simulink model "hopperDesign"  (R2023b)
settings: Solver=VariableStepAuto  StartTime=0.0  StopTime=10.0  RelTol=1e-3
settings Model: Creator=adrnf  LastModifiedBy=adrnf

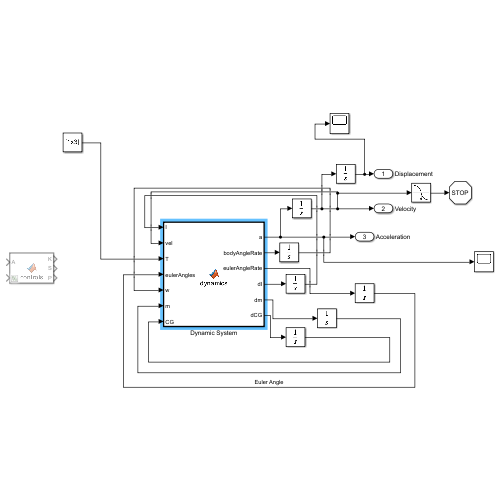
[thumbnail: Simulink's stored preview of the top-level diagram]
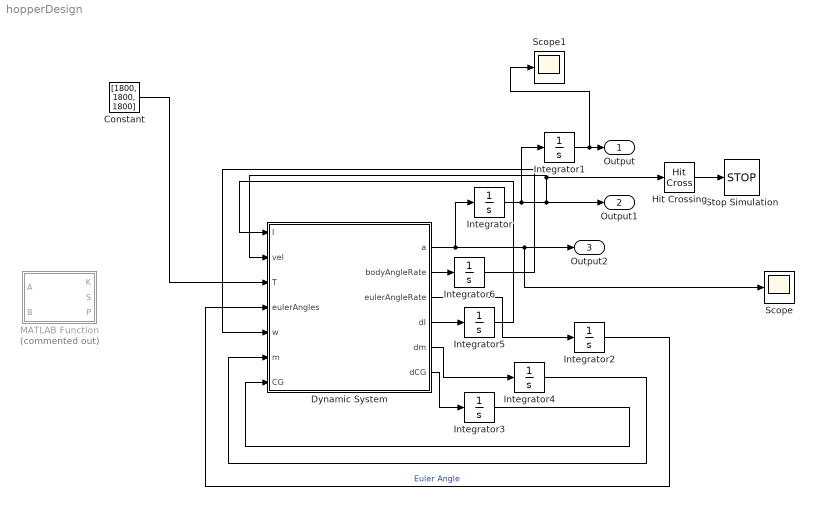
== system hopperDesign ==
  Constant : Constant  Value=[1800, 1800, 1800]
  Dynamic System : MATLAB Function  TreatAsAtomicUnit=on
  Hit Crossing : HitCross  HitCrossingDirection=falling
  Integrator : Integrator  InitialCondition=[0,0,0]
  Integrator1 : Integrator  InitialCondition=[0,0,0]
  Integrator2 : Integrator  InitialCondition=[0;0;0]
  Integrator3 : Integrator  InitialCondition=[5, 0, 0]
  Integrator4 : Integrator  InitialCondition=190
  Integrator5 : Integrator  InitialCondition=[27.920, 0, 0; 0, 27.960, 0; 0, 0, 7.87870]
  Integrator6 : Integrator  InitialCondition=[0,0,0]
  MATLAB Function : MATLAB Function  Commented=on  TreatAsAtomicUnit=on
  Scope : Scope
  Scope1 : Scope
  Stop Simulation : Stop
  Output : Outport  SignalName=Displacement
  Output1 : Outport  Port=2  SignalName=Velocity
  Output2 : Outport  Port=3  SignalName=Acceleration
  wires:
  Dynamic System/1(a) -> Integrator/1, Scope/1, Output2/1
  Integrator/1 -> Hit Crossing/1, Dynamic System/2(vel), Output1/1, Integrator1/1
  Hit Crossing/1 -> Stop Simulation/1
  Integrator1/1 -> Scope1/1, Output/1
  Dynamic System/3(eulerAngleRate) -> Integrator2/1
  Integrator2/1 -> Dynamic System/4(eulerAngles)  "Euler Angle"
  Dynamic System/5(dm) -> Integrator4/1
  Integrator4/1 -> Dynamic System/6(m)
  Dynamic System/6(dCG) -> Integrator3/1
  Integrator3/1 -> Dynamic System/7(CG)
  Dynamic System/4(dI) -> Integrator5/1
  Integrator5/1 -> Dynamic System/1(I)
  Dynamic System/2(bodyAngleRate) -> Integrator6/1
  Integrator6/1 -> Dynamic System/5(w)
  Constant/1 -> Dynamic System/3(T)

== matlab function hopperDesign/MATLAB Function ==
  data: A input; K output; B input; S output; P output
function [K, S, P] = controls(A, B)
    
    qx = 0;
    qy = 0;
    qz = 0;
    qd = 0;
    qe = 0;
    qf = 0;
    
    rtx = 0;
    rty = 0;
    rtz = 0;

    Q = diag([qx, qy, qz, qd, qe, qf]);
    R = diag([rtx, rty, rtz]);
    [K, S, P] = lqr(A, B, Q, R);
    
end

== matlab function hopperDesign/Dynamic System ==
  data: I input; vel input; T input; eulerAngles input; w input; a output; bodyAngleRate output; eulerAngleRate output; dI output; m input; dm output; CG input; dCG output
function [a, bodyAngleRate, eulerAngleRate, dI, dm, dCG]  = dynamics(I, vel, T, eulerAngles, w, m, CG)
    %
    % Inputs: param - Rocket parameters (Dry mass, moment of inertiam cg)
    %         T - Thrust Vector 
    %         w - angular velocity vector
    % Outputs: a - acceleration vector
    %          wd - angular acceleration vector

    Isp = 190;

    engineCG = [10, 0, 0]; % Location of engine in body-fixed axis
    Ixx = I(1,1);
    Iyy = I(2,2);
    Izz = I(3,3);

    vx = vel(1);
    vy = vel(2);
    vz = vel(3);

    Fpx = T(1);
    Fpy = T(2);
    Fpz = T(3);
   
    p = w(1);
    q = w(2);
    r = w(3);
    
    phi = eulerAngles(1);
    theta = eulerAngles(2);
    psi = eulerAngles(3);

    ge = [0; 0; -9.81]; % Acceleration vector due to gravity in Earth-fixed (m/s^2)
    
    % Earth-fixed to Body Fixed Transformation Matrix
    Tbe = [cos(theta)*cos(phi), sin(phi)*sin(theta)*cos(psi) - cos(phi)*sin(psi), cos(phi)*sin(theta)*cos(phi) + sin(phi)*sin(psi);
           cos(theta)*sin(psi), sin(phi)*sin(theta)*sin(psi) + cos(phi)*cos(psi), cos(phi)*sin(theta)*cos(psi) - sin(phi)*cos(psi);
           -sin(theta), sin(phi)*cos(theta), cos(phi)*cos(theta)];

    gb = Tbe * ge;

    ax = Fpx/m + gb(1) - (q*vz - r*vy); % Acceleration in bodyX
    ay = Fpy/m + gb(2) - (r*vx - r*vz); % Acceleration in bodyY
    az = Fpz/m + gb(3) - (p*vy - q*vx); % Acceleration in bodyZ
        
    a = [ax,ay,az]; % Acceleration Vector
    
    diffCG = CG - engineCG;
    moments = [diffCG(2)*T(3)-diffCG(3)*T(2), diffCG(3)*T(1) - diffCG(1)*T(3), diffCG(1)*T(2) - diffCG(2)*T(1)];

    pDot = (moments(1) - (q*r*(Iyy-Izz)))/Ixx;
    qDot = (moments(2) - (p*r*(Ixx - Iyy)))/Iyy;
    rDot = (moments(3) - (p*q*(Ixx - Iyy)))/Izz;
    
    bodyAngleRate = [pDot, qDot, rDot];

    eulerAngleRate = [1, sin(phi)*tan(theta), cos(phi)*tan(theta);
                      0, cos(phi), -sin(phi);
                      0, sin(phi)/cos(theta), cos(phi)/cos(theta)] * w; % From MATLAB
    
    % Update mass
    dI = [-(diffCG(2)^2 + diffCG(3)^2)*T(1)/Isp, 0, 0;
          0, -(diffCG(1)^2 + diffCG(3)^2)*T(2)/Isp, 0;
          0, 0, -(diffCG(1)^2 + diffCG(2)^2)*T(3)/Isp];
    dm = -norm(T)/Isp;
    dCG = [-0.1, 0, 0];




    % % Linearising Control System
    % syms x y z vx vy vz d e f dd ed fd
    % 
    % g = [ vx;
    %       vy;
    %       vz;
    %       ax;
    %       ay;
    %       az;
    %       dd;
    %       ed;
    %       fd;
    %       ddd;
    %       edd;
    %       fdd;
    %       ]



end
